simulink library "SleepingBeautyBtc"  (R2022b)
settings: Solver=VariableStepAuto  StartTime=0.0  StopTime=10.0  RelTol=1e-3
undefined symbols (not defined in the file or in its folder): Row
libraries: TuneVar x8, TOP x3, SetDsm x2, AudioStats x1, FeaturePath x1, HandyTextFile x1, RTC x1
settings Model: Creator=yp1048186  LastModifiedBy=kl13806
settings SolverCC: AlgebraicLoopSolver=TrustRegion
settings DebuggingCC: UnconnectedInputMsg=warning  UnconnectedOutputMsg=warning  UnconnectedLineMsg=warning  SFMachineParentedDataDiag=warning
settings ModelReferenceCC: EnableRefExpFcnMdlSchedulingChecks=on
settings RTWCC: DLArmComputeVersion=19.05

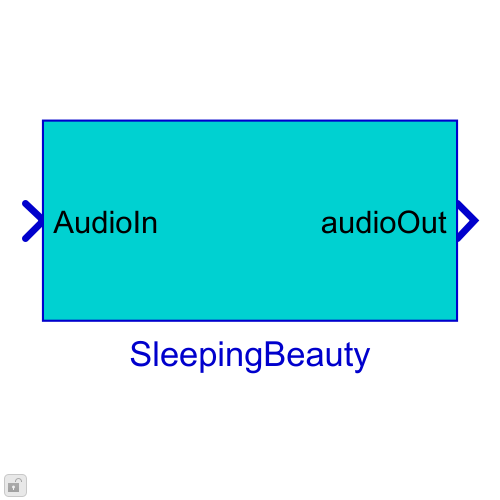
[thumbnail: Simulink's stored preview of the top-level diagram]
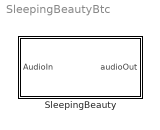
== system SleepingBeautyBtc ==
  SleepingBeauty : Subsystem  mask(Blocklib SleepingBeauty){Config=[], FeatureName=SleepingBeauty}
      mask prompts: Config "SleepingBeautyConfig"; FeatureName "Feature path name:"
      mask help:
      | This block is to be used in conjunction with the Balance block.
      |
      | For the Channel to Ramper Map, enter any of the following values:
      | 1 - left channel
      | 2 - right channel
      | 3 - center channel
      | 4 - mono channel
      | -1 - unused channel (will esentially be muted)
      | (For headrest speakers, choose a seat-centric ramper, i.e. Left Seat Left Ear and Left Seat Right Ear would both be considered "Left content", receiving a 1).
      |
      | Silent Extreme Mutes Bass: Check this box if the intention is for mono channels to be muted upon Silent Extreme
      |
      | If this block is being used in a multi-instance application, be sure to give independent names in each instance's mask.
      mask init:
      | blkh=gcbh;
      | Config=BTConfig.Assert(blkh,Config);
      | 
      | SleepingBeautyMask.Init(blkh);
      | 
      | % Set boundary conditions
      | rampRateBounds = [5,50000];
      | rampTimeBounds = [1,3000];
      | 
      | BTConfig.InitSetFeatureIfPresent(blkh,'FeatureName');
      | Config.Validate();
      mask Callback Config: BTConfig.CallbackHideIfPresent(gcbh,{'FeatureName'});
      mask TypeOptions FeatureName: FeaturePath/FeatureName

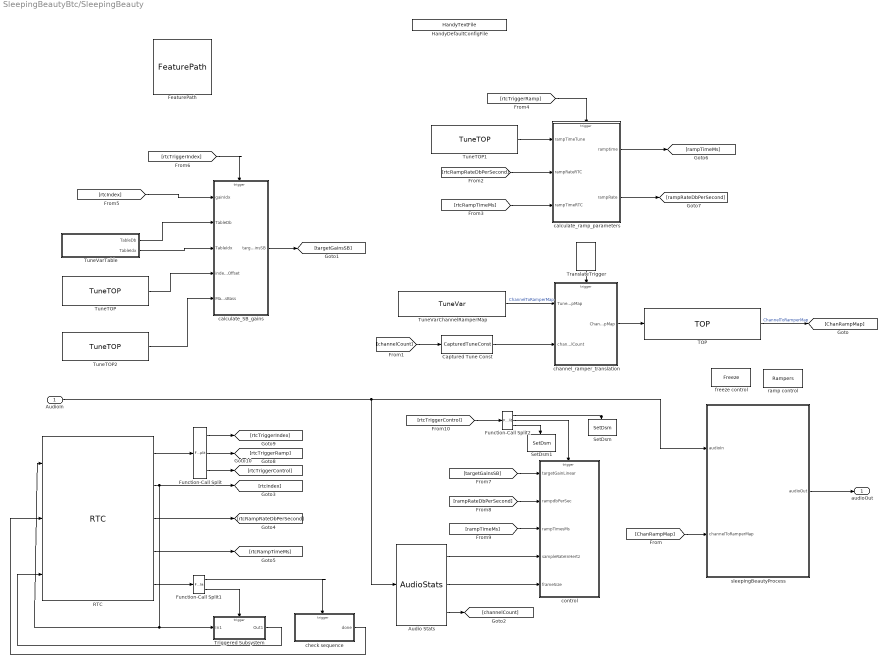
== system SleepingBeautyBtc/SleepingBeauty ==
  AudioIn : Inport
  Audio Stats : AudioStats/AudioStats  DoSampleRate=on  TypeSampleRate=Inherit: auto  DoCallRate=off  TypeCallRate=Inherit: auto  DoFrameSize=on  TypeFrameSize=Inherit: auto  DoChannelCount=on  TypeChannelCount=Inherit: auto  DoTaskRateFactor=off  TypeTaskRateFactor=Inherit: auto  MacroNameRoot=AUDIO  MacroNameRootEval='AUDIO'  IsMacroNameEval=off  MacroSampleRate=off  MacroCallRate=off  MacroFrameSize=off  MacroChannelCount=off  MacroTaskRateFactor=off  MacroTaskId=off  ValidateSampleRate=off  ValueSampleRate=[]  ValidateCallRate=off  ValueCallRate=[]  ValidateFrameSize=off  ValueFrameSize=[]  ValidateChannelCount=off  ValueChannelCount=[]  ValidateTaskRateFactor=off  ValueTaskRateFactor=[]
      settings: SourceProductName=Bose Talaria
  Captured Tune Const : TuneVar/CapturedTuneConst  TriggerInit=[155 22 255 58]  Role=Automatic
      settings: SourceProductName=Bose Talaria
  FeaturePath : FeaturePath/FeaturePath  FeatureName=SleepingBeauty  IsGroup=off  GroupNumber=-1  IsModule=off  TriggerInit=[-415 -561 -300 -454]
      settings: SourceProductName=Bose Talaria
  Function-Call Split : FunctionCallSplit  IconShape=distinctive  NumOutputPorts=3  OutputPortLayout=default
  Function-Call Split1 : FunctionCallSplit  IconShape=distinctive  NumOutputPorts=2  OutputPortLayout=default
  Function-Call Split2 : FunctionCallSplit  IconShape=distinctive  NumOutputPorts=3  OutputPortLayout=default
  HandyDefaultConfigFile : HandyTextFile/HandyTextFile  TemplateSource=Config  FileSuffix=Init  OpenDialogOnLoad=off  UseThisBlockName=off  AddGrandParentNamePrefix=off  TheDefaultText=|  ShowInLibBrowser=on
      | % $(FILENAME) Setup model parameters for each "Init" callback (e.g. update diagram)
      | sample_rate_in_hertz = 44100;
      | frame_size = 32;
      | sysin_channel_count = 2;
      settings: SourceProductName=Bose Talaria
  RTC : RTC/RTC  REQ_Priority=RTC_Mask.NormalPriority  RequestAtInit=off  EnableRequest=on  REQElemName1=gain_index  REQElemType1=uint32  REQElemWidth1=1  REQElemInitial1=[]  REQElemName2=ramp_db_per_second  REQElemType2=uint32  REQElemWidth2=1  REQElemInitial2=[]  REQElemName3=ramp_milliseconds  REQElemType3=uint32  REQElemWidth3=1  REQElemInitial3=[]  REQElemType4=uint32  REQElemWidth4=1  REQElemInitial4=[]  REQElemType5=uint32  REQElemWidth5=1  REQElemInitial5=[]  REQElemType6=uint32  REQElemWidth6=1  REQElemInitial6=[]  REQElemType7=uint32  REQElemWidth7=1  REQElemInitial7=[]  REQElemType8=uint32  REQElemWidth8=1  REQElemInitial8=[]  REQElemType9=uint32  REQElemWidth9=1  REQElemInitial9=[]  REQElemType10=uint32  REQElemWidth10=1  REQElemInitial10=[]  EnableResponse=on  EnableRSP_StatusIn=off  RSPElemName1=gain_index  RSPElemType1=uint32  RSPElemWidth1=1  RSPElemType2=uint32  RSPElemWidth2=1  RSPElemType3=uint32  RSPElemWidth3=1  RSPElemType4=uint32  RSPElemWidth4=1  RSPElemType5=uint32  RSPElemWidth5=1  RSPElemType6=uint32  RSPElemWidth6=1  RSPElemType7=uint32  RSPElemWidth7=1  RSPElemType8=uint32  RSPElemWidth8=1  RSPElemType9=uint32  RSPElemWidth9=1  RSPElemType10=uint32  RSPElemWidth10=1  EnableNotification=on  EnableNTF_PrepTrig=off  NTFElemName1=gain_index  NTFElemType1=uint32  NTFElemWidth1=1  NTFElemType2=uint32  NTFElemWidth2=1  NTFElemType3=uint32  NTFElemWidth3=1  NTFElemType4=uint32  NTFElemWidth4=1  NTFElemType5=uint32  NTFElemWidth5=1  NTFElemType6=uint32  NTFElemWidth6=1  NTFElemType7=uint32  NTFElemWidth7=1  NTFElemType8=uint32  NTFElemWidth8=1  NTFElemType9=uint32  NTFElemWidth9=1  NTFElemType10=uint32  NTFElemWidth10=1  MaskMessageName=Set
      settings: SourceProductName=Bose Talaria
  SetDsm : SetDsm/SetDsm  DataStoreName=Freeze  Value=uint32(1)
      settings: SourceProductName=Bose Talaria
  SetDsm1 : SetDsm/SetDsm  DataStoreName=Freeze  Value=uint32(0)
      settings: SourceProductName=Bose Talaria
  TOP : TOP/TOP  TriggerInit=[555 -30 785 30]  TopName=ChannelToRamperMap  DataType=single  BankNumber=0  PreOverlay=false  PostOverlay=false  Role=Automatic
      settings: SourceProductName=Bose Talaria
  TranslateTrigger : TuneVar/TranslateTrigger  TriggerInit=[421 -160 459 -105]
      settings: SourceProductName=Bose Talaria
  Triggered Subsystem : Subsystem  TreatAsAtomicUnit=on
  TuneTOP : TuneVar/TuneTOP  Description=Defines the index at which the index is at the center, i.e. neither towards the left nor the right sides.  TriggerInit=[-595 -93 -425 -37]  TopName=Offset  TuneName=Offset  DataType=single  TunabilityNumber=1  MinValue=[]  MaxValue=[]  BankNumber=0  PreOverlay=false  PostOverlay=false  UseSameName=on  MaskValue=Config.DefaultOffset
      settings: SourceProductName=Bose Talaria
  TuneTOP1 : TuneVar/TuneTOP  TriggerInit=[135 -393 305 -337]  TopName=RampTime  TuneName=RampTime  DataType=single  TunabilityNumber=1  MinValue=[]  MaxValue=[]  BankNumber=0  PreOverlay=false  PostOverlay=false  UseSameName=on  MaskValue=30
      settings: SourceProductName=Bose Talaria
  TuneTOP2 : TuneVar/TuneTOP  Description=Defines the index at which the index is at the center, i.e. neither towards the left nor the right sides.  TriggerInit=[-595 17 -425 73]  TopName=MutesBass  TuneName=MutesBass  DataType=single  TunabilityNumber=1  MinValue=[]  MaxValue=[]  BankNumber=0  PreOverlay=false  PostOverlay=false  UseSameName=on  MaskValue=Config.DefaultSilentExtremeMutesBass
      settings: SourceProductName=Bose Talaria
  TuneVarChannelRamperMap : TuneVar/TuneVar  TuneName=ChannelToRamperMap  SpecifyMaxSize=off  VariableDim=1 (Row)  MaxSize=[1 1]  TunabilityNumber=1  MinValue=[]  MaxValue=[]  TriggerInit=[70 -65 280 -15]  MaskValue=Config.ChanToRampMap
      settings: SourceProductName=Bose Talaria
  TuneVarTable : Subsystem
  calculate_SB_gains : MATLAB Function  TreatAsAtomicUnit=on  mask{MaskNumRampers=Config.NumRampers}
  calculate_ramp_parameters : MATLAB Function  TreatAsAtomicUnit=on
  channel_ramper_translation : MATLAB Function  TreatAsAtomicUnit=on  mask{MaskNumRampers=Config.NumRampers}
  check sequence : MATLAB Function  TreatAsAtomicUnit=on  mask{MaskNumRampers=Config.NumRampers}
  control : MATLAB Function  TreatAsAtomicUnit=on  mask{MaskNumRampers=Config.NumRampers}
  freeze control : DataStoreMemory  DataStoreName=Freeze  ShowAdditionalParam=off  OutDataTypeStr=uint32
  ramp control : DataStoreMemory  DataStoreName=Rampers  ReadBeforeWriteMsg=warning  WriteAfterWriteMsg=warning  WriteAfterReadMsg=warning  InitialValue=Config.DlgRamperInit  ShowAdditionalParam=off  OutDataTypeStr=Bus: rgain_bus
  sleepingBeautyProcess : MATLAB Function  TreatAsAtomicUnit=on  mask{MaskNumRampers=Config.NumRampers}
  audioOut : Outport
  wires:
  RTC/1 -> Function-Call Split/1
  RTC/4 -> [rtcRampTimeMs]
  RTC/3 -> [rtcRampRateDbPerSecond]
  AudioIn/1 -> Audio Stats/1, sleepingBeautyProcess/1(audioIn)
  TranslateTrigger/1 -> channel_ramper_translation/Trigger
  TuneVarChannelRamperMap/1 -> channel_ramper_translation/1(TuneChanRampMap)  "ChannelToRamperMap"
  channel_ramper_translation/1(ChanRampMap) -> TOP/1
  TOP/1 -> [ChanRampMap]  "ChannelToRamperMap"
  [ChanRampMap] -> sleepingBeautyProcess/2(channelToRamperMap)
  TuneVarTable/1(TableDb) -> calculate_SB_gains/2(TableDb)
  TuneVarTable/2(TableIdx) -> calculate_SB_gains/3(TableIdx)
  TuneTOP/1 -> calculate_SB_gains/4(indexOffset)
  calculate_SB_gains/1(targetGainsSB) -> [targetGainsSB]
  Audio Stats/3 -> [channelCount]
  [channelCount] -> Captured Tune Const/1
  Captured Tune Const/1 -> channel_ramper_translation/2(channelCount)
  [rtcRampRateDbPerSecond] -> calculate_ramp_parameters/2(rampRateRTC)
  TuneTOP1/1 -> calculate_ramp_parameters/1(rampTimeTune)
  [rtcRampTimeMs] -> calculate_ramp_parameters/3(rampTimeRTC)
  calculate_ramp_parameters/1(ramptime) -> [rampTimeMs]
  calculate_ramp_parameters/2(rampRate) -> [rampRateDbPerSecond]
  RTC/2 -> Triggered Subsystem/1(In1), RTC/1, [rtcIndex]
  Function-Call Split/2 -> [rtcTriggerRamp]
  Function-Call Split/3 -> [rtcTriggerControl]
  Function-Call Split/1 -> [rtcTriggerIndex]
  [rtcTriggerRamp] -> calculate_ramp_parameters/Trigger
  [rtcIndex] -> calculate_SB_gains/1(gainIdx)
  [rtcTriggerIndex] -> calculate_SB_gains/Trigger
  [targetGainsSB] -> control/1(targetGainLinear)
  [rampRateDbPerSecond] -> control/2(rampdbPerSec)
  [rampTimeMs] -> control/3(rampTimesMs)
  [rtcTriggerControl] -> Function-Call Split2/1
  Audio Stats/1 -> control/4(sampleRateInHertz)
  Audio Stats/2 -> control/5(frameSize)
  sleepingBeautyProcess/1(audioOut) -> audioOut/1
  RTC/5 -> Function-Call Split1/1
  Function-Call Split1/1 -> check sequence/Trigger
  Function-Call Split1/2 -> Triggered Subsystem/Trigger
  check sequence/1(done) -> RTC/2
  Triggered Subsystem/1(Out1) -> RTC/3
  TuneTOP2/1 -> calculate_SB_gains/5(MaskSilentExtremeMutesBass)
  Function-Call Split2/1 -> SetDsm/Trigger
  Function-Call Split2/2 -> control/Trigger
  Function-Call Split2/3 -> SetDsm1/Trigger

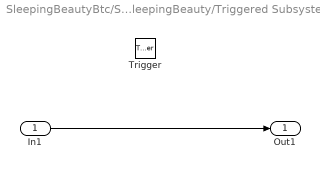
== system SleepingBeautyBtc/SleepingBeauty/Triggered Subsystem ==
  In1 : Inport
  Trigger : TriggerPort  TriggerType=function-call  VariantControl=Variant
  Out1 : Outport
  wires:
  In1/1 -> Out1/1

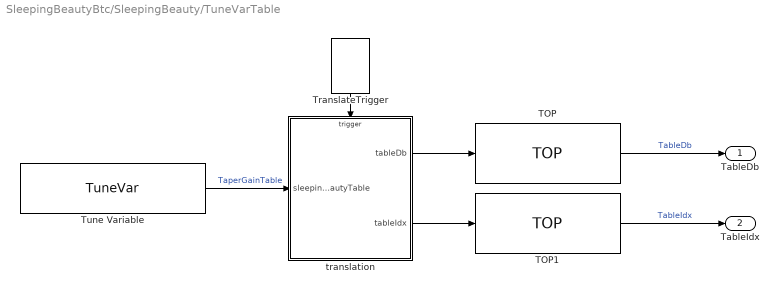
== system SleepingBeautyBtc/SleepingBeauty/TuneVarTable ==
  TOP : TOP/TOP  TriggerInit=[90 240 235 300]  TopName=TableDb  DataType=single  BankNumber=0  PreOverlay=false  PostOverlay=false  Role=Automatic
      settings: SourceProductName=Bose Talaria
  TOP1 : TOP/TOP  TriggerInit=[90 310 235 370]  TopName=TableIdx  DataType=single  BankNumber=0  PreOverlay=false  PostOverlay=false  Role=Automatic
      settings: SourceProductName=Bose Talaria
  TranslateTrigger : TuneVar/TranslateTrigger  TriggerInit=[-54 155 -16 210]
      settings: SourceProductName=Bose Talaria
  Tune Variable : TuneVar/TuneVar  TuneName=TaperGainTable  SpecifyMaxSize=on  VariableDim=1 (Row)  MaxSize=[30 2]  TunabilityNumber=1  MinValue=[]  MaxValue=[]  TriggerInit=[-365 280 -180 330]  MaskValue=Config.DefaultTaperGainTable
      settings: SourceProductName=Bose Talaria
  translation : MATLAB Function  TreatAsAtomicUnit=on
  TableDb : Outport
  TableIdx : Outport  Port=2
  wires:
  TOP/1 -> TableDb/1  "TableDb"
  TranslateTrigger/1 -> translation/Trigger
  Tune Variable/1 -> translation/1(sleepingBeautyTable)  "TaperGainTable"
  translation/1(tableDb) -> TOP/1
  translation/2(tableIdx) -> TOP1/1
  TOP1/1 -> TableIdx/1  "TableIdx"

== matlab function SleepingBeautyBtc/SleepingBeauty/TuneVarTable/translation ==
  data: tableDb output; sleepingBeautyTable input; tableIdx output
  events: trigger input FUNCTION_CALL_EVENT
function [tableDb, tableIdx]  = fcn(sleepingBeautyTable)
%#codegen

% Set up the size and datatype of our TOP outputs:
maxTableSize = numel(sleepingBeautyTable.Value) / 2;
idxType = 'uint8';
idxStorageType = 'uint32';
dbType = 'single';
tableIdx = zeros(1,maxTableSize,idxStorageType);
tableDb = zeros(1,maxTableSize,dbType);

% separate the pairs into their index and value components
givenPairs = sleepingBeautyTable.Size(1);
indices = sleepingBeautyTable.Value(1:givenPairs,1);
values = sleepingBeautyTable.Value(1:givenPairs,2);

% then sort and ignore duplicates
[cleanIdx,map] = unique(indices);

% Validate input sizes
numPairs = numel(map);
argName='sleepingBeautyTable';

% Validate: enough data?
if (numPairs < 2)
    TranslateError('%s must have at least 2 index pairs. Encounted value with only %f pairs\n', argName, numPairs);
end

% Validate: Highest index still below 255?
if (cleanIdx(1) < 0 || cleanIdx(end) > intmax(idxType))
    TranslateError('%s out of range table index %f encountered. Index must be between 0 and %d.\n',argName,cleanIdx(end),intmax(idxType));
end

% fill in the table buffer with provided pairs
tableIdx(1:numPairs) = cleanIdx(1:numPairs);
tableDb(1:numPairs) = values(map(1:numPairs));

% fill the rest of the table buffer with the last entry
remainingPairs = numel(map)+1:maxTableSize;
tableIdx(remainingPairs) = tableIdx(numPairs);
tableDb(remainingPairs) =  tableDb(numPairs);

end

== matlab function SleepingBeautyBtc/SleepingBeauty/sleepingBeautyProcess ==
  data: audioIn input; audioOut output; channelToRamperMap input; MaskNumRampers parameter; Rampers data_store_memory; Freeze data_store_memory
function audioOut  = sleepingBeautyProcess(audioIn, channelToRamperMap, ... % inputs
    MaskNumRampers)  % parameters

% Applies the Left and Right gains to the respective channels via multiple
%   rampers
% Inputs:
%  audioIn: Input audio
%  channelToRamperMap: Input channels mapped to their corresponding ramper.
%  MaskNumRampers: Number of rampers (set in the Mask file) = 4

% Data Store objects (registered in "Edit Data" dialog)
global Rampers;
global Freeze;

% Figure out the frame size, channel count and number of rampers
[frameSize, ~] = size(audioIn);

% set the size and datatype of the output buffer
audioOut = coder.nullcopy(audioIn);

%   Every channel needs a ramper, but every ramper does not need to be on a
%   channel necessarily.
for ramper = 1:MaskNumRampers
    % Get the gains
    gain = Rampers(ramper).currentGain;
    rampCoeffMultipliers = ones(1, frameSize, 'single');
    if (Freeze(1) == false)
        if (Rampers(ramper).frameCount == 0)
            % The ramp is finished. Stop ramping and SNAP to the target
            gain = Rampers(ramper).targetGain;
        else
            % The ramp is *NOT* frozen or done: gain is moving
            k = Rampers(ramper).rampCoeff;
            rampCoeffMultipliers = (k * rampCoeffMultipliers) .^ (1:frameSize);
            Rampers(ramper).frameCount = Rampers(ramper).frameCount - 1;
        end
    end
    
    % Apply the gains to the corresponding channels via the Mask parameter
    % and tuneTop paramter "channelToRamperMap".  
    currentChannelGroup = find(channelToRamperMap == ramper);
    for ch = 1:numel(currentChannelGroup)
        audioOut(:,currentChannelGroup(ch)) = (gain * rampCoeffMultipliers)' .* audioIn(:,currentChannelGroup(ch));
    end
    Rampers(ramper).currentGain = gain * rampCoeffMultipliers(end);
end

% If ramper value of -1 is encountered, this indicates an unused channel.
% Assign values of zero to all samples of these channels.
unusedChannelGroup = find(channelToRamperMap == -1);
for unusedCh = 1:numel(unusedChannelGroup)
    audioOut(:,unusedChannelGroup(unusedCh)) = 0;
end

== matlab function SleepingBeautyBtc/SleepingBeauty/calculate_SB_gains ==
  data: gainIdx input; targetGainsSB output; TableDb input; TableIdx input; indexOffset input; MaskNumRampers parameter; MaskSilentExtremeMutesBass input
  events: trigger input FUNCTION_CALL_EVENT
function targetGainsSB = Calculate_SB_Gains(gainIdx, TableDb,...
    TableIdx, indexOffset,MaskNumRampers, MaskSilentExtremeMutesBass)

% Computes the gains for the L, R, C Mono channel groups.  
% Based on the gainIdx, we will:
%     1. Set specific speakers to mute, if the gain index is 
%     extreme (i.e. either 0 or 255)
%     2. Begin a gain-tapering function on the speakers, if the
%     gain index is approaching 0 or 255 (i.e. taper the speaker gains
%     beginning with the last few clicks of the gain index)

%  Set target gains to ones
j = uint8(1);
cut_linear = single(0.0);

targetGainsSB = coder.nullcopy(ones(1, MaskNumRampers,'single'));
gainIdx = single(gainIdx);
    
% Find the left and the right gains
% Based on the SB table, the dB value of the index is calculated
while (j <= numel(TableIdx))
    if (gainIdx <= TableIdx(j))
        if (j <= 1)  % first indexed value is linearly interpolated to zero
            if (TableIdx(j))
                percent = gainIdx / TableIdx(j);
            else
                percent = single(1);
            end
            cut_linear = percent * 10 ^ (TableDb(j) / 20);
        else         % other values are interpolated in db space
            lastIdx = single(TableIdx(j-1));
            percent = (gainIdx - lastIdx) / (TableIdx(j) - lastIdx);
            cut_linear = 10 ^ (((percent * (TableDb(j) - TableDb(j-1))) + TableDb(j-1)) / 20);
        end
        break;
    else
        j = j + 1;
    end
end

% Assign left and right Gain Values to headrest speakers (TAPERING)
if (gainIdx - indexOffset) > 0 % Left speakers attenuated
    left = single(cut_linear);
    right = single(1);
    center = left;
    mono = center;
    
    % % If we're extreme, make the cut complete
    if (abs(gainIdx - indexOffset) >= (indexOffset-1))
        left = single(0);
        center = single(0);
    end
else                           % Right speakers attenuated 
    right = single(cut_linear);
    left = single(1);
    center = right;  
    mono = center;
    
        % % If we're extreme, make the cut complete
    if (abs(gainIdx - indexOffset) >= (indexOffset-1))
        right = single(0);
        center = single(0);
    end
end

% Mute the mono channels if we're extreme and if it's checked in the mask
if (abs(gainIdx - indexOffset) >= (indexOffset-1)) && (MaskSilentExtremeMutesBass) 
    mono = single(0);
end

% Write gains to targetGains 
targetGainsSB(1) = left;
targetGainsSB(2) = right;
targetGainsSB(3) = center;
targetGainsSB(4) = mono;

end

== matlab function SleepingBeautyBtc/SleepingBeauty/calculate_ramp_parameters ==
  data: rampTimeTune input; ramptime output; rampRateRTC input; rampTimeRTC input; rampRate output; rampTimeBounds parameter; rampRateBounds parameter
  events: trigger input FUNCTION_CALL_EVENT
function [ramptime, rampRate]  = calculate_ramp_parameters(...
    rampTimeTune, rampRateRTC,rampTimeRTC, ... % inputs
    rampTimeBounds, rampRateBounds) % parameters

% Ramp time and rate are provided to the block through SB RTC messages
% However in case neither of them are provided, the block will use the 
% default ramp time given in the tune variables.

    ramptime = single(rampTimeTune);
    rampRate = single(0);

    if (rampRateRTC)
        rampRate = single(rampRateRTC);
        rampRate = max(rampRateBounds(1), rampRate);
        rampRate = min(rampRateBounds(2), rampRate);
    end
    if (rampTimeRTC)
        ramptime = single(rampTimeRTC);
    end
    ramptime = max(rampTimeBounds(1), ramptime);
    ramptime = min(rampTimeBounds(2), ramptime);
end

== matlab function SleepingBeautyBtc/SleepingBeauty/control ==
  data: targetGainLinear input; rampdbPerSec input; rampTimesMs input; sampleRateInHertz input; frameSize input; MaskNumRampers parameter; Rampers data_store_memory
  events: trigger input FUNCTION_CALL_EVENT
function control(...
     targetGainLinear, rampdbPerSec, rampTimesMs, sampleRateInHertz, ...
     frameSize, ... % inputs
     MaskNumRampers) % parameters
%#codegen
% CONTROL LOGIC:
% Shift of 'balance' between the 'Right' and 'Left' channel groups is
% achieved by multiplying the corresponding 'cut' or 'boost' gain. As the
% index increases from 0, the balance shifts from left to right.
% rampdbPerSec takes precidence:
%   If dbPerSec has a non-zero value then any ramp_times_ms values are
%   ignored and the dbPerSec is used to determine ramper timing.
% Inputs:
%   targetGainLinear: Indicates the gain (in linear scale) which needs to
%       be applied to the audio. Gain values can be mapped to the ramper
%       configuration.
%   rampTimeMs: Indicates the time in milliseconds in which the gain of the
%       rampers must change from their current to target values.
%   rampdbPerSecond: Indicates the rate in dB/second at which the gain of the
%       rampers must change from their current to target values. If this
%       value is non-zero, it is used to compute the ramp time and
%       'rampTimeMs' is discarded (if specified).
%   rgain_SILENT_GAIN: Parameter defined in the initFcn callback.

% Control Data:
%   Freeze(1) freezes the processing during this control operation
%   Rampers(1) is the ramper for the left speaker
%   Rampers(2) is the ramper for the right speaker
%   Rampers(3) is the ramper for the center speaker
%   Rampers(4) is the ramper for the mono speaker

global Rampers;

rgain_SILENT_GAIN = RgainBusUtil.GetSilentGainLinear();

% Step 1: FREEZE the gain ramper so that we can perform calculations based
% on the current gain value. This step now done externally on canvas

% Step 2: Nudge the gain values a bit if they are sitting at zero.
% When this control set goes live, ensure that the current gain will move.
% If current gain is zero, replace with a value very close to zero. What we
% really want is a value which is on the edge of perception - not too small
% or large. If the value is too small, we'll waste some of our ramp time
% in perceived silence. If the value is too large, the audio will lurch
% into perceptability at the start of the ramp.
% UPDATE: This will now loop over 4 rampers

currentGainLinear = zeros(1,MaskNumRampers,'single');
for i = 1:MaskNumRampers
    currentGainLinear(i) = max(Rampers(i).currentGain, rgain_SILENT_GAIN);
    targetGainLinear(i) = max(targetGainLinear(i), rgain_SILENT_GAIN);
end

% Step 3a: If a slope in dB/second is provided, ignore the ramp time
% and instead calculate a new ramp time that matches the slope.
rampMs = zeros(1,MaskNumRampers,'single');
if (rampdbPerSec)
    currentGainDb = 20*log10(currentGainLinear);
    targetGainDb = 20*log10(targetGainLinear);
    diff = abs(currentGainDb - targetGainDb);
    rampMs = diff / single(rampdbPerSec) * 1000;
else
    rampMs(:) = single(rampTimesMs);
end
    
% Step 3b: QUANTIZE the desired ramp time to our FrameSize. Also retrieve 
% the whole number of frames required to best match requested ramp time.
% Ensure that at least one frame is used. The frame size will therefore
% determine the steepest ramp (i.e. within one frame you can go anywhere).
quantumMs = 1000 * frameSize / sampleRateInHertz;
numFrames = rampMs / quantumMs;
numFrames = max (1, ceil(numFrames));
quantizedRampTimeMs = numFrames * quantumMs;

% UPDATE: Loop over 4 rampers now (L, R, C, and Mono)
for ramper=1:MaskNumRampers
    % In order to have the desired ramp time, the slope must vary dependent
    % on the gain differencebetween target and current value.
    % Ramper's coefficient is therefore calculated as follows:
    %
    %   TargetGain = CurrentGain *( RampCoef ^ (Fs*RampTime_ms/1000) )
    %
    % therefore...
    %
    %                     log(TargetGain/CurrentGain)
    %   log(RampCoef) = ------------------------------
    %                        Fs*(RampTime_ms/1000)
    %
    factor = log( targetGainLinear(ramper) / currentGainLinear(ramper) );
    RampCoef = double(exp(factor / (sampleRateInHertz * quantizedRampTimeMs(ramper) / 1000)));
    
    % Output control signals
    Rampers(ramper).frameCount  = int32(numFrames(ramper));    
    Rampers(ramper).targetGain  = targetGainLinear(ramper);
    Rampers(ramper).rampCoeff = single(RampCoef);
    Rampers(ramper).currentGain = currentGainLinear(ramper);
end
% unfreeze the gain. This step now done externally on canvas

== matlab function SleepingBeautyBtc/SleepingBeauty/channel_ramper_translation ==
  data: ChanRampMap output; TuneChanRampMap input; channelCount input; MaskNumRampers parameter
  events: trigger input FUNCTION_CALL_EVENT
function ChanRampMap = fcn(TuneChanRampMap, channelCount, ... %Inputs
    MaskNumRampers) % Parameters

% Function that verifies channel-to-ramper map is valid
% Takes channelRamperMap and channelCount as inputs, and 
% number of rampers as a parameter
argName = 'SleepingBeauty';

% Ensure each channel is present in the map
inputMapWidth = numel(TuneChanRampMap.Value);
if (inputMapWidth ~= channelCount)
   error(['Error in %s : Channel-to-ramper map width [%d] does not match number of ',...
       'audio channels [%d]. Make sure all channels are assigned ',...
       'to either the left or right groups.'], argName, inputMapWidth, ...
       channelCount);
end

% Verifies if each channel is assigned to one of the 5 possible rampers.

if (numel(unique(TuneChanRampMap.Value)) > (MaskNumRampers + 1))
    error(['Error in [%s] : Atleast 1 channel has been assigned to the incorrect group.' ...
        'Group numbers assigned to channels in the Channel-to-ramper '...
        'map should be a number between 1 and [%d], corresponding to one '...
        'of the 3 possible speaker contents .'], argName, MaskNumRampers);        
end

% Verify that a value of 0 was not incorrectly entered as a ramper
if (sum(TuneChanRampMap.Value == 0) > 0)
   error(['Error in [%s] : Valid ramper values for the channel to '...
       'ramper map must be between 1 and [%d}, or "-1" to indicate an '... 
       'unused channel .'], argName), MaskNumRampers;
end

ChanRampMap = int32(TuneChanRampMap.Value);

== matlab function SleepingBeautyBtc/SleepingBeauty/check sequence ==
  data: done output; Rampers data_store_memory; MaskNumRampers parameter
  events: trigger input FUNCTION_CALL_EVENT
function done = GetCompletedSequence(MaskNumRampers)
%  Function that checks whether all channels have completed their ramp to 
% target gain.
% If so, send out TRUE to RTC

global Rampers;

% Assume the work is complete until proven otherwise
done = true;

for i=1:MaskNumRampers
   if (Rampers(i).targetGain ~= Rampers(i).currentGain)
       done = false; % just proved otherwise
       break;
   end
end
